simulink model "throttle_error_unit_test"  (R2024a)
settings: Solver=VariableStepAuto  StartTime=0.0  StopTime=10.0  RelTol=1e-3
settings Model: Creator=lucap  LastModifiedBy=lucap

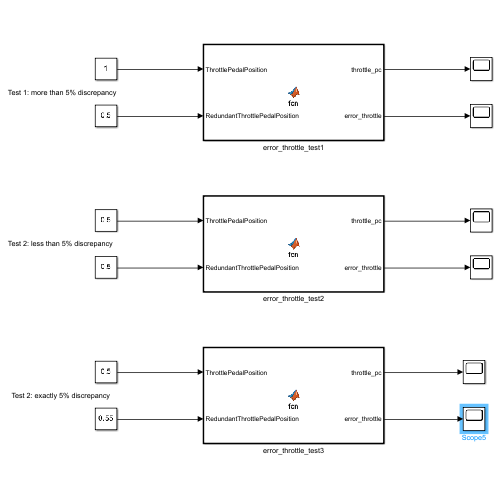
[thumbnail: Simulink's stored preview of the top-level diagram]
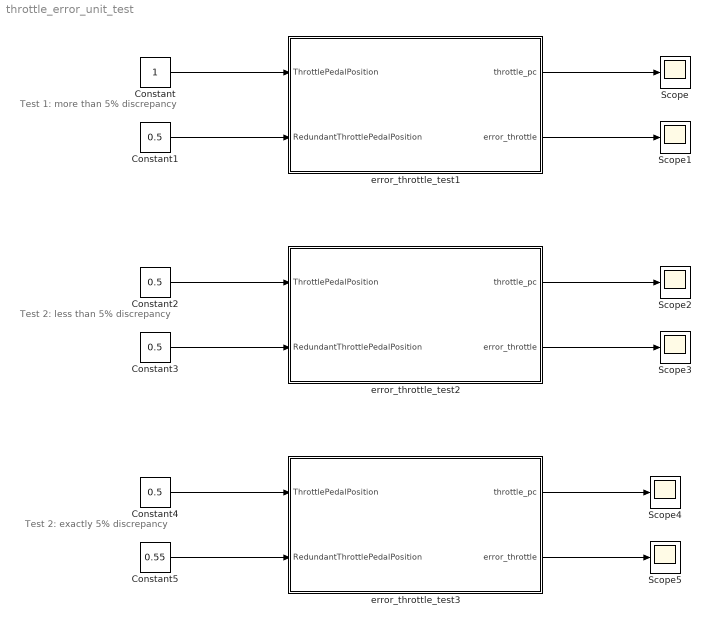
== system throttle_error_unit_test ==
  note: Test 1: more than 5% discrepancy
  note: Test 2: less than 5% discrepancy
  note: Test 2: exactly 5% discrepancy
  Constant : Constant
  Constant{1..4} (4 alike) : Constant  Value=0.5
  Constant5 : Constant  Value=0.55
  Scope{,1..5} (6 alike) : Scope
  error_throttle_test1 : MATLAB Function  TreatAsAtomicUnit=on
  error_throttle_test2 : MATLAB Function  TreatAsAtomicUnit=on
  error_throttle_test3 : MATLAB Function  TreatAsAtomicUnit=on
  wires:
  Constant/1 -> error_throttle_test1/1(ThrottlePedalPosition)
  Constant1/1 -> error_throttle_test1/2(RedundantThrottlePedalPosition)
  Constant2/1 -> error_throttle_test2/1(ThrottlePedalPosition)
  Constant3/1 -> error_throttle_test2/2(RedundantThrottlePedalPosition)
  Constant4/1 -> error_throttle_test3/1(ThrottlePedalPosition)
  Constant5/1 -> error_throttle_test3/2(RedundantThrottlePedalPosition)
  error_throttle_test1/1(throttle_pc) -> Scope/1
  error_throttle_test1/2(error_throttle) -> Scope1/1
  error_throttle_test2/1(throttle_pc) -> Scope2/1
  error_throttle_test2/2(error_throttle) -> Scope3/1
  error_throttle_test3/1(throttle_pc) -> Scope4/1
  error_throttle_test3/2(error_throttle) -> Scope5/1

== matlab function throttle_error_unit_test/error_throttle_test1 ==
  data: throttle_pc output; ThrottlePedalPosition input; error_throttle output; RedundantThrottlePedalPosition input
function [throttle_pc, error_throttle]  = fcn(ThrottlePedalPosition, RedundantThrottlePedalPosition)

diff = abs(ThrottlePedalPosition - RedundantThrottlePedalPosition);
diff = round(diff * 1000) / 1000; % avoid matlab numerical errors

if diff > 0.05
    error_throttle = boolean(1);
    throttle_pc = single(-1);
else
    error_throttle = boolean(0);
    throttle_pc = single(ThrottlePedalPosition);
end

== matlab function throttle_error_unit_test/error_throttle_test3 ==
  data: throttle_pc output; ThrottlePedalPosition input; error_throttle output; RedundantThrottlePedalPosition input
function [throttle_pc, error_throttle]  = fcn(ThrottlePedalPosition, RedundantThrottlePedalPosition)

diff = abs(ThrottlePedalPosition - RedundantThrottlePedalPosition);
diff = round(diff * 1000) / 1000; % avoid matlab numerical errors

if diff > 0.05
    error_throttle = boolean(1);
    throttle_pc = single(-1);
else
    error_throttle = boolean(0);
    throttle_pc = single(ThrottlePedalPosition);
end

== matlab function throttle_error_unit_test/error_throttle_test2 ==
  data: throttle_pc output; ThrottlePedalPosition input; error_throttle output; RedundantThrottlePedalPosition input
function [throttle_pc, error_throttle]  = fcn(ThrottlePedalPosition, RedundantThrottlePedalPosition)

diff = abs(ThrottlePedalPosition - RedundantThrottlePedalPosition);
diff = round(diff * 1000) / 1000; % avoid matlab numerical errors

if diff > 0.05
    error_throttle = boolean(1);
    throttle_pc = single(-1);
else
    error_throttle = boolean(0);
    throttle_pc = single(ThrottlePedalPosition);
end
